simulink model "Open_Loop_Simulation"  (R2021a)
settings: Solver=VariableStepAuto  StartTime=0.0  StopTime=tsim  RelTol=1e-3
undefined symbols (not defined in the file or in its folder): A1, a1, A2, a2, A3, a3, A4, a4, Adlin, Alin, Bdlin, Blin, C, Cdlin, g, gamma1, gamma2, k1, k2, m, n, sat_hmax, sat_hmin, sat_vmax, sigma_b, Ts, v01, v02, x0, xd0
libraries: simulink x4
settings Model: Creator=aperodou  LastModifiedBy=Arthur
settings SolverCC: AlgebraicLoopSolver=TrustRegion
settings DebuggingCC: SFMachineParentedDataDiag=warning

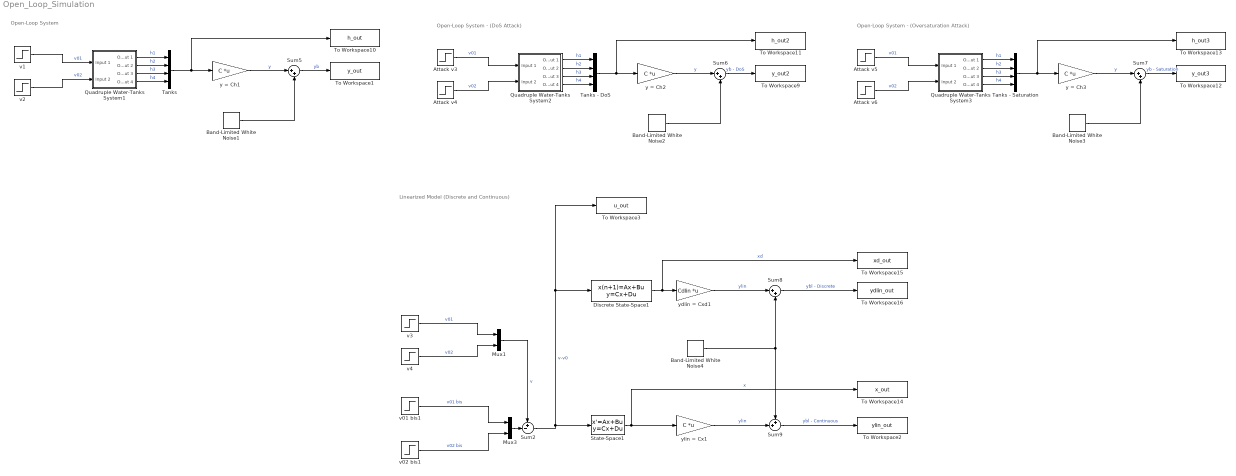
== system Open_Loop_Simulation ==
  note: Linearized Model
      | (Discrete and Continuous)
  note: Open-Loop System
  note: Open-Loop System - (DoS Attack)
  note: Open-Loop System - (Oversaturation Attack)
  Attack v3 : Step  Time=0  After=0  SampleTime=0
  Attack v4 : Step  Time=0  After=0  SampleTime=0
  Attack v5 : Step  Time=0  After=sat_vmax  SampleTime=0
  Attack v6 : Step  Time=0  After=sat_vmax  SampleTime=0
  Band-Limited White Noise{1..4} (4 alike) : simulink/Sources/Band-Limited White Noise  Cov=[ sigma_b sigma_b ]  Ts=Ts  seed=[23341]
  Discrete State-Space1 : DiscreteStateSpace  A=Adlin  B=Bdlin  C=eye(n)  D=zeros(n,m)  InitialCondition=xd0  SampleTime=Ts
  Mux1 : Mux  Inputs=2
  Mux3 : Mux  Inputs=2
  Quadruple Water-Tanks System1 : Subsystem
  Quadruple Water-Tanks System2 : Subsystem
  Quadruple Water-Tanks System3 : Subsystem
  State-Space1 : StateSpace  A=Alin  B=Blin  C=eye(n)  D=zeros(n,m)  InitialCondition=x0
  Sum2 : Sum  Inputs=+-|  SaturateOnIntegerOverflow=on
  Sum{5..8} (4 alike) : Sum  Inputs=|++  SaturateOnIntegerOverflow=on
  Sum9 : Sum  Inputs=++|  SaturateOnIntegerOverflow=on
  Tanks : Mux
  Tanks - DoS : Mux
  Tanks - Saturation : Mux
  To Workspace1 : ToWorkspace  VariableName=y_out  SaveFormat=Timeseries  SampleTime=-1
  To Workspace10 : ToWorkspace  VariableName=h_out  SaveFormat=Timeseries  SampleTime=-1
  To Workspace11 : ToWorkspace  VariableName=h_out2  SaveFormat=Timeseries  SampleTime=-1
  To Workspace12 : ToWorkspace  VariableName=y_out3  SaveFormat=Timeseries  SampleTime=-1
  To Workspace13 : ToWorkspace  VariableName=h_out3  SaveFormat=Timeseries  SampleTime=-1
  To Workspace14 : ToWorkspace  VariableName=x_out  SaveFormat=Timeseries  SampleTime=-1
  To Workspace15 : ToWorkspace  VariableName=xd_out  SaveFormat=Timeseries  SampleTime=-1
  To Workspace16 : ToWorkspace  VariableName=ydlin_out  SaveFormat=Timeseries  SampleTime=-1
  To Workspace2 : ToWorkspace  VariableName=ylin_out  SaveFormat=Timeseries  SampleTime=-1
  To Workspace3 : ToWorkspace  VariableName=u_out  SaveFormat=Timeseries  SampleTime=-1
  To Workspace9 : ToWorkspace  VariableName=y_out2  SaveFormat=Timeseries  SampleTime=-1
  v01 bis1 : Step  Time=0  After=v01  SampleTime=0
  v02 bis1 : Step  Time=0  After=v02  SampleTime=0
  v1 : Step  Time=0  After=v01  SampleTime=0
  v2 : Step  Time=0  After=v02  SampleTime=0
  v3 : Step  Time=0  After=v01  SampleTime=0
  v4 : Step  Time=0  After=v02  SampleTime=0
  y = Ch1 : Gain  Gain=C  Multiplication=Matrix(K*u) (u vector)
  y = Ch2 : Gain  Gain=C  Multiplication=Matrix(K*u) (u vector)
  y = Ch3 : Gain  Gain=C  Multiplication=Matrix(K*u) (u vector)
  ydlin = Cxd1 : Gain  Gain=Cdlin  Multiplication=Matrix(K*u) (u vector)
  ylin = Cx1 : Gain  Gain=C  Multiplication=Matrix(K*u) (u vector)
  wires:
  y = Ch1/1 -> Sum5/1  "y"
  Quadruple Water-Tanks System1/2(Output 2) -> Tanks/2  "h2"
  Band-Limited White Noise1/1 -> Sum5/2
  Quadruple Water-Tanks System1/4(Output 4) -> Tanks/4  "h4"
  Sum5/1 -> To Workspace1/1  "yb"
  Quadruple Water-Tanks System1/1(Output 1) -> Tanks/1  "h1"
  v1/1 -> Quadruple Water-Tanks System1/1(Input 1)  "v01"
  Quadruple Water-Tanks System1/3(Output 3) -> Tanks/3  "h3"
  Tanks/1 -> To Workspace10/1, y = Ch1/1
  v2/1 -> Quadruple Water-Tanks System1/2(Input 2)  "v02"
  Attack v4/1 -> Quadruple Water-Tanks System2/2(Input 2)  "v02"
  Attack v3/1 -> Quadruple Water-Tanks System2/1(Input 1)  "v01"
  Quadruple Water-Tanks System2/3(Output 3) -> Tanks - DoS/3  "h3"
  Sum6/1 -> To Workspace9/1  "yb - DoS"
  Tanks - DoS/1 -> To Workspace11/1, y = Ch2/1
  Quadruple Water-Tanks System2/1(Output 1) -> Tanks - DoS/1  "h1"
  Quadruple Water-Tanks System2/2(Output 2) -> Tanks - DoS/2  "h2"
  y = Ch2/1 -> Sum6/1  "y"
  Band-Limited White Noise2/1 -> Sum6/2
  Quadruple Water-Tanks System2/4(Output 4) -> Tanks - DoS/4  "h4"
  Attack v6/1 -> Quadruple Water-Tanks System3/2(Input 2)  "v02"
  Attack v5/1 -> Quadruple Water-Tanks System3/1(Input 1)  "v01"
  Quadruple Water-Tanks System3/3(Output 3) -> Tanks - Saturation/3  "h3"
  Sum7/1 -> To Workspace12/1  "yb - Saturation"
  Tanks - Saturation/1 -> To Workspace13/1, y = Ch3/1
  Quadruple Water-Tanks System3/1(Output 1) -> Tanks - Saturation/1  "h1"
  Quadruple Water-Tanks System3/2(Output 2) -> Tanks - Saturation/2  "h2"
  y = Ch3/1 -> Sum7/1  "y"
  Band-Limited White Noise3/1 -> Sum7/2
  Quadruple Water-Tanks System3/4(Output 4) -> Tanks - Saturation/4  "h4"
  ydlin = Cxd1/1 -> Sum8/1  "ylin"
  State-Space1/1 -> To Workspace14/1, ylin = Cx1/1  "x"
  ylin = Cx1/1 -> Sum9/2  "ylin"
  Sum9/1 -> To Workspace2/1  "ybl - Continuous"
  Sum8/1 -> To Workspace16/1  "ybl - Discrete"
  Mux1/1 -> Sum2/1  "v"
  Mux3/1 -> Sum2/2
  Band-Limited White Noise4/1 -> Sum9/1, Sum8/2
  Discrete State-Space1/1 -> To Workspace15/1, ydlin = Cxd1/1  "xd"
  v3/1 -> Mux1/1  "v01"
  v02 bis1/1 -> Mux3/2  "v02 bis"
  v4/1 -> Mux1/2  "v02"
  v01 bis1/1 -> Mux3/1  "v01 bis"
  Sum2/1 -> State-Space1/1, To Workspace3/1, Discrete State-Space1/1  "v-v0"

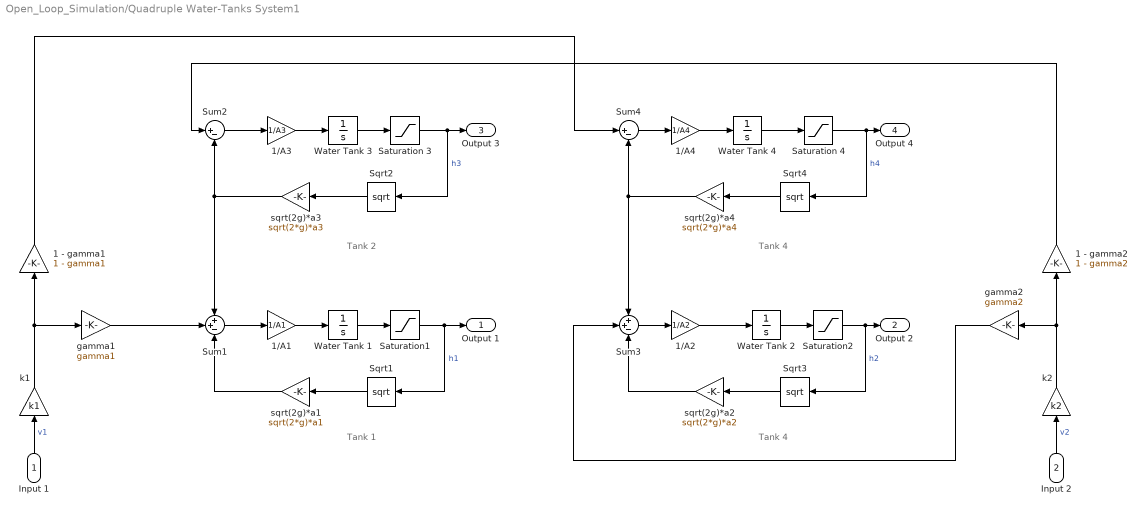
== system Open_Loop_Simulation/Quadruple Water-Tanks System1 ==
  note: Tank 1
  note: Tank 2
  note: Tank 4
  note: Tank 4
  Input 1 : Inport
  Input 2 : Inport  Port=2
  1 - gamma1 : Gain  Gain=1 - gamma1  SaturateOnIntegerOverflow=on  OutDataTypeStr=Inherit: Same as input  ParamDataTypeStr=Inherit: Same as input
  1 - gamma2 : Gain  Gain=1 - gamma2  SaturateOnIntegerOverflow=on  OutDataTypeStr=Inherit: Same as input  ParamDataTypeStr=Inherit: Same as input
  1/A1 : Gain  Gain=1/A1  SaturateOnIntegerOverflow=on  OutDataTypeStr=Inherit: Same as input  ParamDataTypeStr=Inherit: Same as input
  1/A2 : Gain  Gain=1/A2  SaturateOnIntegerOverflow=on  OutDataTypeStr=Inherit: Same as input  ParamDataTypeStr=Inherit: Same as input
  1/A3 : Gain  Gain=1/A3  SaturateOnIntegerOverflow=on  OutDataTypeStr=Inherit: Same as input  ParamDataTypeStr=Inherit: Same as input
  1/A4 : Gain  Gain=1/A4  SaturateOnIntegerOverflow=on  OutDataTypeStr=Inherit: Same as input  ParamDataTypeStr=Inherit: Same as input
  Saturation 3 : Saturate  UpperLimit=sat_hmax  LowerLimit=sat_hmin
  Saturation 4 : Saturate  UpperLimit=sat_hmax  LowerLimit=sat_hmin
  Saturation1 : Saturate  UpperLimit=sat_hmax  LowerLimit=sat_hmin
  Saturation2 : Saturate  UpperLimit=sat_hmax  LowerLimit=sat_hmin
  Sqrt{1..4} (4 alike) : Sqrt  SaturateOnIntegerOverflow=on
  Sum1 : Sum  Inputs=++-  SaturateOnIntegerOverflow=on
  Sum2 : Sum  Inputs=|+-  SaturateOnIntegerOverflow=on
  Sum3 : Sum  Inputs=++-  SaturateOnIntegerOverflow=on
  Sum4 : Sum  Inputs=|+-  SaturateOnIntegerOverflow=on
  Water Tank {1..4} (4 alike) : Integrator
  gamma1 : Gain  Gain=gamma1  SaturateOnIntegerOverflow=on  OutDataTypeStr=Inherit: Same as input  ParamDataTypeStr=Inherit: Same as input
  gamma2 : Gain  Gain=gamma2  SaturateOnIntegerOverflow=on  OutDataTypeStr=Inherit: Same as input  ParamDataTypeStr=Inherit: Same as input
  k1 : Gain  Gain=k1  SaturateOnIntegerOverflow=on  OutDataTypeStr=Inherit: Same as input  ParamDataTypeStr=Inherit: Same as input
  k2 : Gain  Gain=k2  SaturateOnIntegerOverflow=on  OutDataTypeStr=Inherit: Same as input  ParamDataTypeStr=Inherit: Same as input
  sqrt(2g)*a1 : Gain  Gain=sqrt(2*g)*a1  SaturateOnIntegerOverflow=on  OutDataTypeStr=Inherit: Same as input  ParamDataTypeStr=Inherit: Same as input
  sqrt(2g)*a2 : Gain  Gain=sqrt(2*g)*a2  SaturateOnIntegerOverflow=on  OutDataTypeStr=Inherit: Same as input  ParamDataTypeStr=Inherit: Same as input
  sqrt(2g)*a3 : Gain  Gain=sqrt(2*g)*a3  SaturateOnIntegerOverflow=on  OutDataTypeStr=Inherit: Same as input  ParamDataTypeStr=Inherit: Same as input
  sqrt(2g)*a4 : Gain  Gain=sqrt(2*g)*a4  SaturateOnIntegerOverflow=on  OutDataTypeStr=Inherit: Same as input  ParamDataTypeStr=Inherit: Same as input
  Output 1 : Outport  VectorParamsAs1DForOutWhenUnconnected=off
  Output 2 : Outport  Port=2  VectorParamsAs1DForOutWhenUnconnected=off
  Output 3 : Outport  Port=3  VectorParamsAs1DForOutWhenUnconnected=off
  Output 4 : Outport  Port=4  VectorParamsAs1DForOutWhenUnconnected=off
  wires:
  Saturation2/1 -> Sqrt3/1, Output 2/1  "h2"
  Water Tank 2/1 -> Saturation2/1
  Water Tank 4/1 -> Saturation 4/1
  1/A1/1 -> Water Tank 1/1
  Sqrt2/1 -> sqrt(2g)*a3/1
  Saturation1/1 -> Sqrt1/1, Output 1/1  "h1"
  Water Tank 3/1 -> Saturation 3/1
  sqrt(2g)*a3/1 -> Sum2/2, Sum1/1
  sqrt(2g)*a4/1 -> Sum4/2, Sum3/1
  Saturation 3/1 -> Sqrt2/1, Output 3/1  "h3"
  Saturation 4/1 -> Sqrt4/1, Output 4/1  "h4"
  1/A4/1 -> Water Tank 4/1
  Water Tank 1/1 -> Saturation1/1
  Sum1/1 -> 1/A1/1
  Sqrt3/1 -> sqrt(2g)*a2/1
  k1/1 -> 1 - gamma1/1, gamma1/1
  Sqrt4/1 -> sqrt(2g)*a4/1
  k2/1 -> 1 - gamma2/1, gamma2/1
  Sum4/1 -> 1/A4/1
  gamma1/1 -> Sum1/2
  1 - gamma1/1 -> Sum4/1
  Input 2/1 -> k2/1  "v2"
  sqrt(2g)*a2/1 -> Sum3/3
  sqrt(2g)*a1/1 -> Sum1/3
  Sum2/1 -> 1/A3/1
  gamma2/1 -> Sum3/2
  1 - gamma2/1 -> Sum2/1
  1/A2/1 -> Water Tank 2/1
  Sum3/1 -> 1/A2/1
  1/A3/1 -> Water Tank 3/1
  Sqrt1/1 -> sqrt(2g)*a1/1
  Input 1/1 -> k1/1  "v1"

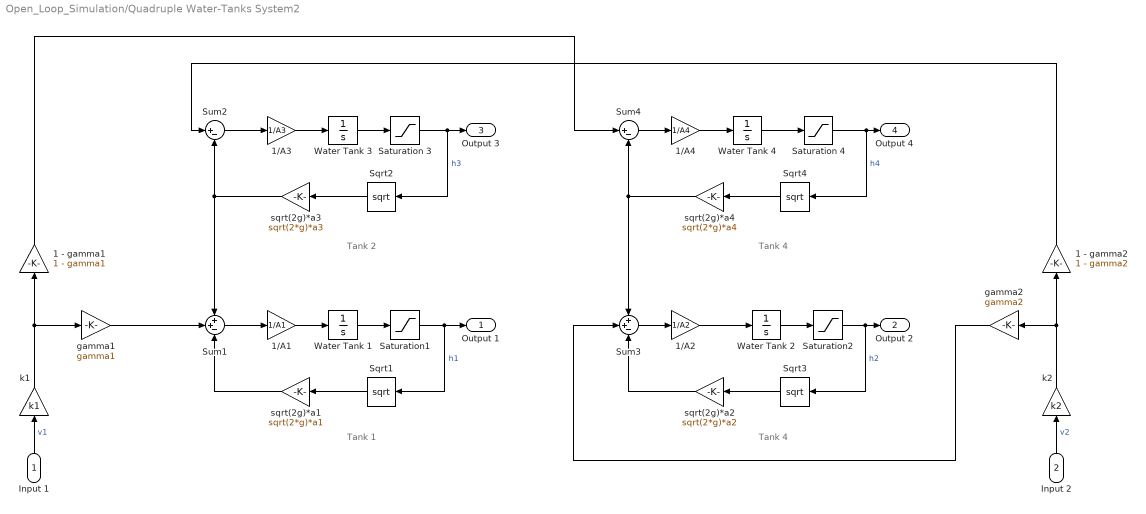
== system Open_Loop_Simulation/Quadruple Water-Tanks System2 ==
  note: Tank 1
  note: Tank 2
  note: Tank 4
  note: Tank 4
  Input 1 : Inport
  Input 2 : Inport  Port=2
  1 - gamma1 : Gain  Gain=1 - gamma1  SaturateOnIntegerOverflow=on  OutDataTypeStr=Inherit: Same as input  ParamDataTypeStr=Inherit: Same as input
  1 - gamma2 : Gain  Gain=1 - gamma2  SaturateOnIntegerOverflow=on  OutDataTypeStr=Inherit: Same as input  ParamDataTypeStr=Inherit: Same as input
  1/A1 : Gain  Gain=1/A1  SaturateOnIntegerOverflow=on  OutDataTypeStr=Inherit: Same as input  ParamDataTypeStr=Inherit: Same as input
  1/A2 : Gain  Gain=1/A2  SaturateOnIntegerOverflow=on  OutDataTypeStr=Inherit: Same as input  ParamDataTypeStr=Inherit: Same as input
  1/A3 : Gain  Gain=1/A3  SaturateOnIntegerOverflow=on  OutDataTypeStr=Inherit: Same as input  ParamDataTypeStr=Inherit: Same as input
  1/A4 : Gain  Gain=1/A4  SaturateOnIntegerOverflow=on  OutDataTypeStr=Inherit: Same as input  ParamDataTypeStr=Inherit: Same as input
  Saturation 3 : Saturate  UpperLimit=sat_hmax  LowerLimit=sat_hmin
  Saturation 4 : Saturate  UpperLimit=sat_hmax  LowerLimit=sat_hmin
  Saturation1 : Saturate  UpperLimit=sat_hmax  LowerLimit=sat_hmin
  Saturation2 : Saturate  UpperLimit=sat_hmax  LowerLimit=sat_hmin
  Sqrt{1..4} (4 alike) : Sqrt  SaturateOnIntegerOverflow=on
  Sum1 : Sum  Inputs=++-  SaturateOnIntegerOverflow=on
  Sum2 : Sum  Inputs=|+-  SaturateOnIntegerOverflow=on
  Sum3 : Sum  Inputs=++-  SaturateOnIntegerOverflow=on
  Sum4 : Sum  Inputs=|+-  SaturateOnIntegerOverflow=on
  Water Tank {1..4} (4 alike) : Integrator
  gamma1 : Gain  Gain=gamma1  SaturateOnIntegerOverflow=on  OutDataTypeStr=Inherit: Same as input  ParamDataTypeStr=Inherit: Same as input
  gamma2 : Gain  Gain=gamma2  SaturateOnIntegerOverflow=on  OutDataTypeStr=Inherit: Same as input  ParamDataTypeStr=Inherit: Same as input
  k1 : Gain  Gain=k1  SaturateOnIntegerOverflow=on  OutDataTypeStr=Inherit: Same as input  ParamDataTypeStr=Inherit: Same as input
  k2 : Gain  Gain=k2  SaturateOnIntegerOverflow=on  OutDataTypeStr=Inherit: Same as input  ParamDataTypeStr=Inherit: Same as input
  sqrt(2g)*a1 : Gain  Gain=sqrt(2*g)*a1  SaturateOnIntegerOverflow=on  OutDataTypeStr=Inherit: Same as input  ParamDataTypeStr=Inherit: Same as input
  sqrt(2g)*a2 : Gain  Gain=sqrt(2*g)*a2  SaturateOnIntegerOverflow=on  OutDataTypeStr=Inherit: Same as input  ParamDataTypeStr=Inherit: Same as input
  sqrt(2g)*a3 : Gain  Gain=sqrt(2*g)*a3  SaturateOnIntegerOverflow=on  OutDataTypeStr=Inherit: Same as input  ParamDataTypeStr=Inherit: Same as input
  sqrt(2g)*a4 : Gain  Gain=sqrt(2*g)*a4  SaturateOnIntegerOverflow=on  OutDataTypeStr=Inherit: Same as input  ParamDataTypeStr=Inherit: Same as input
  Output 1 : Outport  VectorParamsAs1DForOutWhenUnconnected=off
  Output 2 : Outport  Port=2  VectorParamsAs1DForOutWhenUnconnected=off
  Output 3 : Outport  Port=3  VectorParamsAs1DForOutWhenUnconnected=off
  Output 4 : Outport  Port=4  VectorParamsAs1DForOutWhenUnconnected=off
  wires:
  Saturation2/1 -> Sqrt3/1, Output 2/1  "h2"
  Water Tank 2/1 -> Saturation2/1
  Water Tank 4/1 -> Saturation 4/1
  1/A1/1 -> Water Tank 1/1
  Sqrt2/1 -> sqrt(2g)*a3/1
  Saturation1/1 -> Sqrt1/1, Output 1/1  "h1"
  Water Tank 3/1 -> Saturation 3/1
  sqrt(2g)*a3/1 -> Sum2/2, Sum1/1
  sqrt(2g)*a4/1 -> Sum4/2, Sum3/1
  Saturation 3/1 -> Sqrt2/1, Output 3/1  "h3"
  Saturation 4/1 -> Sqrt4/1, Output 4/1  "h4"
  1/A4/1 -> Water Tank 4/1
  Water Tank 1/1 -> Saturation1/1
  Sum1/1 -> 1/A1/1
  Sqrt3/1 -> sqrt(2g)*a2/1
  k1/1 -> 1 - gamma1/1, gamma1/1
  Sqrt4/1 -> sqrt(2g)*a4/1
  k2/1 -> 1 - gamma2/1, gamma2/1
  Sum4/1 -> 1/A4/1
  gamma1/1 -> Sum1/2
  1 - gamma1/1 -> Sum4/1
  Input 2/1 -> k2/1  "v2"
  sqrt(2g)*a2/1 -> Sum3/3
  sqrt(2g)*a1/1 -> Sum1/3
  Sum2/1 -> 1/A3/1
  gamma2/1 -> Sum3/2
  1 - gamma2/1 -> Sum2/1
  1/A2/1 -> Water Tank 2/1
  Sum3/1 -> 1/A2/1
  1/A3/1 -> Water Tank 3/1
  Sqrt1/1 -> sqrt(2g)*a1/1
  Input 1/1 -> k1/1  "v1"

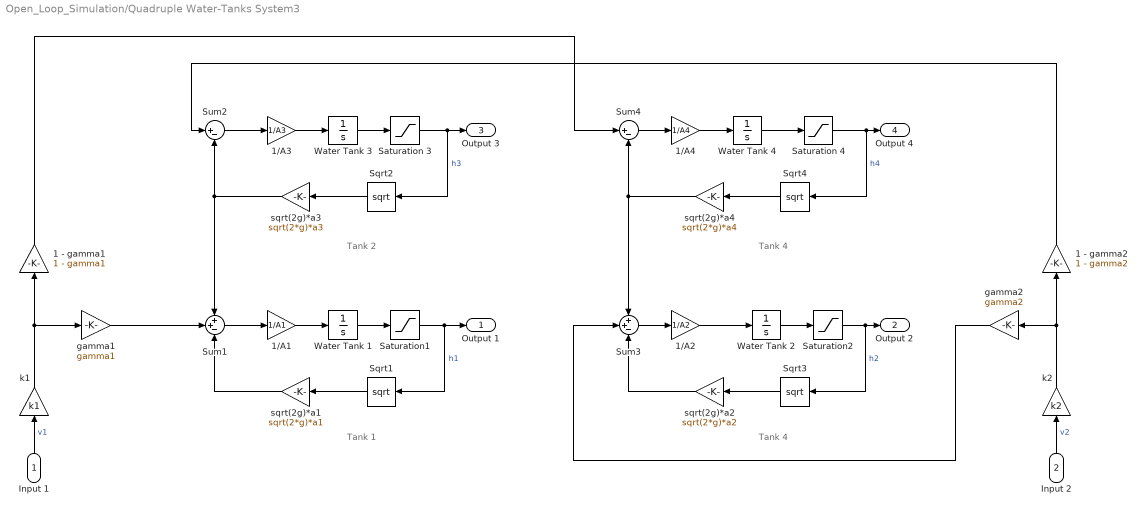
== system Open_Loop_Simulation/Quadruple Water-Tanks System3 ==
  note: Tank 1
  note: Tank 2
  note: Tank 4
  note: Tank 4
  Input 1 : Inport
  Input 2 : Inport  Port=2
  1 - gamma1 : Gain  Gain=1 - gamma1  SaturateOnIntegerOverflow=on  OutDataTypeStr=Inherit: Same as input  ParamDataTypeStr=Inherit: Same as input
  1 - gamma2 : Gain  Gain=1 - gamma2  SaturateOnIntegerOverflow=on  OutDataTypeStr=Inherit: Same as input  ParamDataTypeStr=Inherit: Same as input
  1/A1 : Gain  Gain=1/A1  SaturateOnIntegerOverflow=on  OutDataTypeStr=Inherit: Same as input  ParamDataTypeStr=Inherit: Same as input
  1/A2 : Gain  Gain=1/A2  SaturateOnIntegerOverflow=on  OutDataTypeStr=Inherit: Same as input  ParamDataTypeStr=Inherit: Same as input
  1/A3 : Gain  Gain=1/A3  SaturateOnIntegerOverflow=on  OutDataTypeStr=Inherit: Same as input  ParamDataTypeStr=Inherit: Same as input
  1/A4 : Gain  Gain=1/A4  SaturateOnIntegerOverflow=on  OutDataTypeStr=Inherit: Same as input  ParamDataTypeStr=Inherit: Same as input
  Saturation 3 : Saturate  UpperLimit=sat_hmax  LowerLimit=sat_hmin
  Saturation 4 : Saturate  UpperLimit=sat_hmax  LowerLimit=sat_hmin
  Saturation1 : Saturate  UpperLimit=sat_hmax  LowerLimit=sat_hmin
  Saturation2 : Saturate  UpperLimit=sat_hmax  LowerLimit=sat_hmin
  Sqrt{1..4} (4 alike) : Sqrt  SaturateOnIntegerOverflow=on
  Sum1 : Sum  Inputs=++-  SaturateOnIntegerOverflow=on
  Sum2 : Sum  Inputs=|+-  SaturateOnIntegerOverflow=on
  Sum3 : Sum  Inputs=++-  SaturateOnIntegerOverflow=on
  Sum4 : Sum  Inputs=|+-  SaturateOnIntegerOverflow=on
  Water Tank {1..4} (4 alike) : Integrator
  gamma1 : Gain  Gain=gamma1  SaturateOnIntegerOverflow=on  OutDataTypeStr=Inherit: Same as input  ParamDataTypeStr=Inherit: Same as input
  gamma2 : Gain  Gain=gamma2  SaturateOnIntegerOverflow=on  OutDataTypeStr=Inherit: Same as input  ParamDataTypeStr=Inherit: Same as input
  k1 : Gain  Gain=k1  SaturateOnIntegerOverflow=on  OutDataTypeStr=Inherit: Same as input  ParamDataTypeStr=Inherit: Same as input
  k2 : Gain  Gain=k2  SaturateOnIntegerOverflow=on  OutDataTypeStr=Inherit: Same as input  ParamDataTypeStr=Inherit: Same as input
  sqrt(2g)*a1 : Gain  Gain=sqrt(2*g)*a1  SaturateOnIntegerOverflow=on  OutDataTypeStr=Inherit: Same as input  ParamDataTypeStr=Inherit: Same as input
  sqrt(2g)*a2 : Gain  Gain=sqrt(2*g)*a2  SaturateOnIntegerOverflow=on  OutDataTypeStr=Inherit: Same as input  ParamDataTypeStr=Inherit: Same as input
  sqrt(2g)*a3 : Gain  Gain=sqrt(2*g)*a3  SaturateOnIntegerOverflow=on  OutDataTypeStr=Inherit: Same as input  ParamDataTypeStr=Inherit: Same as input
  sqrt(2g)*a4 : Gain  Gain=sqrt(2*g)*a4  SaturateOnIntegerOverflow=on  OutDataTypeStr=Inherit: Same as input  ParamDataTypeStr=Inherit: Same as input
  Output 1 : Outport  VectorParamsAs1DForOutWhenUnconnected=off
  Output 2 : Outport  Port=2  VectorParamsAs1DForOutWhenUnconnected=off
  Output 3 : Outport  Port=3  VectorParamsAs1DForOutWhenUnconnected=off
  Output 4 : Outport  Port=4  VectorParamsAs1DForOutWhenUnconnected=off
  wires:
  Saturation2/1 -> Sqrt3/1, Output 2/1  "h2"
  Water Tank 2/1 -> Saturation2/1
  Water Tank 4/1 -> Saturation 4/1
  1/A1/1 -> Water Tank 1/1
  Sqrt2/1 -> sqrt(2g)*a3/1
  Saturation1/1 -> Sqrt1/1, Output 1/1  "h1"
  Water Tank 3/1 -> Saturation 3/1
  sqrt(2g)*a3/1 -> Sum2/2, Sum1/1
  sqrt(2g)*a4/1 -> Sum4/2, Sum3/1
  Saturation 3/1 -> Sqrt2/1, Output 3/1  "h3"
  Saturation 4/1 -> Sqrt4/1, Output 4/1  "h4"
  1/A4/1 -> Water Tank 4/1
  Water Tank 1/1 -> Saturation1/1
  Sum1/1 -> 1/A1/1
  Sqrt3/1 -> sqrt(2g)*a2/1
  k1/1 -> 1 - gamma1/1, gamma1/1
  Sqrt4/1 -> sqrt(2g)*a4/1
  k2/1 -> 1 - gamma2/1, gamma2/1
  Sum4/1 -> 1/A4/1
  gamma1/1 -> Sum1/2
  1 - gamma1/1 -> Sum4/1
  Input 2/1 -> k2/1  "v2"
  sqrt(2g)*a2/1 -> Sum3/3
  sqrt(2g)*a1/1 -> Sum1/3
  Sum2/1 -> 1/A3/1
  gamma2/1 -> Sum3/2
  1 - gamma2/1 -> Sum2/1
  1/A2/1 -> Water Tank 2/1
  Sum3/1 -> 1/A2/1
  1/A3/1 -> Water Tank 3/1
  Sqrt1/1 -> sqrt(2g)*a1/1
  Input 1/1 -> k1/1  "v1"
